simulink model "simpleTVCRocketModel"  (R2024a)
settings: Solver=ode45  StartTime=0.0  StopTime=15  RelTol=1e-3
PostLoadFcn:
  | VSS_MODE = 0;
undefined symbols (not defined in the file): X, Y, Z
libraries: sm_lib x19, nesl_utility x10, Quintic_Polynomial_Trajectory_Library x3, simulink x1, shared3dof x1, slpidlib x1
(part 2 of 2)

== matlab function simpleTVCRocketModel/MATLAB Function ==
  data: pos input; theta output; waypoint input
function theta = compute_heading_angle(pos, waypoint)
% Computes the angle (in radians) from current position to the waypoint,
% and prints the distance between the two points.
%
% Inputs:
%   pos      - [x, y] vector of current position
%   waypoint - [x, y] vector of target waypoint position
%
% Output:
%   theta    - angle in radians from pos to waypoint (measured from +x axis, counter-clockwise)

% Vector from current position to waypoint
dir = waypoint - pos;

% Compute angle using atan2
theta = atan2(dir(2), dir(1));

% Compute distance
dist = norm(dir);

% Print distance
fprintf('[Heading Angle] Distance to waypoint: %.3f meters\n', dist);

end

== matlab function simpleTVCRocketModel/MATLAB Function2 ==
  data: v_current input; thrust output; v_desired input; mass input; dt input
function thrust = velocityController2D(v_current, v_desired, mass, dt)
%{
#codegen

% Ensure output is always defined

% Declare persistent variables
persistent int_error prev_error
if isempty(int_error)
    int_error = 0;
    prev_error = 0;
end

% Compute current speed
v_mag = norm(v_current);

% Speed error
error = v_desired - v_mag;

% Derivative and integral
d_error = (error - prev_error) / dt;
int_error = int_error + error * dt;

% Controller gains defined in Simulink workspace
Kp = 10;
Ki = 5;
Kd = 2;

% Acceleration command
a_cmd = Kp*error + Ki*int_error + Kd*d_error;

% Direction of thrust (unit vector)
if v_mag > 1e-3
    dir = v_current / v_mag;
else
    dir = [1; 0];  % Default direction
end

% Compute thrust force
thrust = mass * a_cmd * dir;

% Update memory
prev_error = error;
%}
thrust = 20;

== matlab function simpleTVCRocketModel/MATLAB Function3 ==
  data: P0 input; F output; T0 input; hole_diameter input; mdot output; v_exit output
function [F, mdot, v_exit] = estimateRCSForce(P0, T0, hole_diameter)
% Estimates thrust force for choked flow through a small orifice.
%
% Inputs:
%   P0            - Upstream pressure [Pa] (absolute)
%   T0            - Upstream temperature [K]
%   hole_diameter - Diameter of nozzle/orifice [m]
%   gas           - Gas type as string: 'CO2', 'Air', or 'N2'
%
% Outputs:
%   F      - Estimated thrust force [N]
%   mdot   - Estimated mass flow rate [kg/s]
%   v_exit - Estimated exit velocity [m/s]
gas = 'CO2';
% Gas properties
switch upper(gas)
    case 'CO2'
        gamma = 1.3;
        R = 189;      % J/kg·K
    case 'AIR'
        gamma = 1.4;
        R = 287;
    case 'N2'
        gamma = 1.4;
        R = 296;
    otherwise
        error('Unsupported gas: %s. Choose CO2, Air, or N2.', gas);
end

% Constants
Cd = 0.85; % discharge coefficient (typical range: 0.8–1.0)

% Area of the hole
A = pi * (hole_diameter / 2)^2;

% Exit velocity (choked flow assumption)
v_exit = sqrt( (2 * gamma * R * T0) / (gamma + 1) );

% Mass flow rate (choked flow)
mdot = Cd * A * P0 * sqrt( gamma / (R * T0) ) ...
       * ( (2 / (gamma + 1))^((gamma + 1)/(2*(gamma - 1))) );

% Thrust
F = mdot * v_exit;

end
